simulink model "Part_g"  (R2016a)
settings: Solver=VariableStepAuto  StartTime=0.0  StopTime=10.0  RelTol=1e-3
values from neighbouring files (symbols this model uses):
  A = [1,0.00958419619475136,0.0104077383156783,0;0,0.880217654134450,2.02956823954280,0;0,-0.102406711940655,0.862350586928406,0;1,0.00958419619475136,0.0104077383156783,1]    [Project_2.m]
  Ao = A-L*C    [Project_2.m]
  B = [0.0388811995595289;11.5416986681227;10.5268226869341;0.0388811995595289]    [Project_2.m]
  K = place(A,B,[-7,-8,-9,-10])    [Project_2.m]
  L = acker(A',C',PO)'    [Project_2.m]
  Np = 1/N    [Project_2.m]
  x0 = [.2;0;0;0]    [Project_2.m]
settings Model: Creator=ACER  LastModifiedBy=ACER

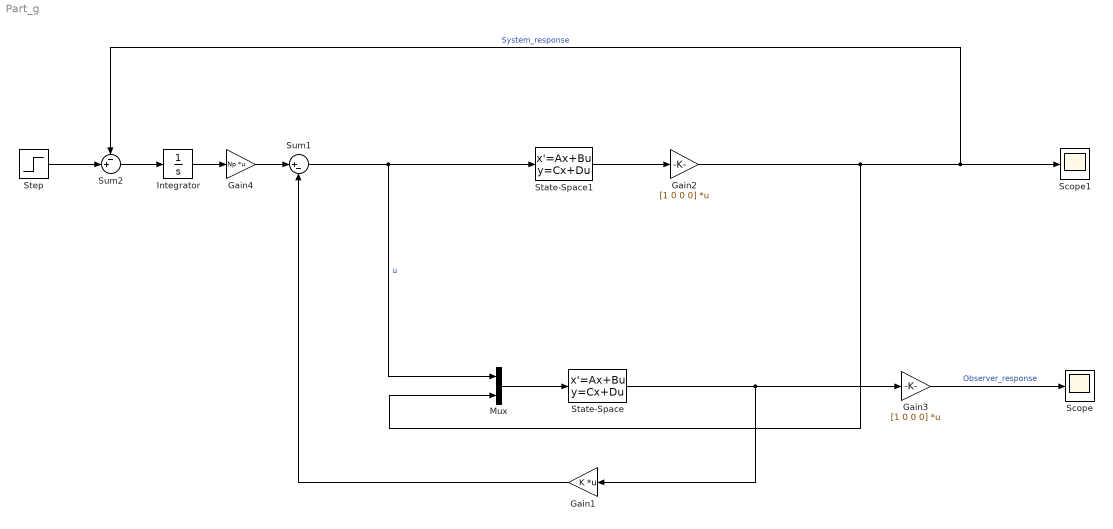
== system Part_g ==
  Gain1 : Gain  Gain=K  Multiplication=Matrix(K*u)
  Gain2 : Gain  Gain=[1 0 0 0]  Multiplication=Matrix(K*u)
  Gain3 : Gain  Gain=[1 0 0 0]  Multiplication=Matrix(K*u)
  Gain4 : Gain  Gain=Np  Multiplication=Matrix(K*u)
  Integrator : Integrator
  Mux : Mux  Inputs=2
  Scope : Scope
  Scope1 : Scope
  State-Space : StateSpace  A=Ao  B=[B L]  C=eye(4)  D=[0 0;0 0;0 0;0 0]  X0=0
  State-Space1 : StateSpace  A=A  B=B  C=eye(4)  D=[0;0;0;0]  X0=x0
  Step : Step  SampleTime=0
  Sum1 : Sum  Inputs=|+-
  Sum2 : Sum  Inputs=-+|
  wires:
  Gain1/1 -> Sum1/2
  Mux/1 -> State-Space/1
  State-Space1/1 -> Gain2/1
  State-Space/1 -> Gain3/1, Gain1/1
  Gain3/1 -> Scope/1  "Observer_response"
  Sum1/1 -> State-Space1/1, Mux/1  "u"
  Integrator/1 -> Gain4/1
  Step/1 -> Sum2/2
  Sum2/1 -> Integrator/1
  Gain2/1 -> Scope1/1, Sum2/1, Mux/2  "System_response"
  Gain4/1 -> Sum1/1
